simulink subsystem "MFTrailerTiresLongitudinal"  (R2023a)
settings: Solver=VariableStepAuto  StartTime=0.0  StopTime=10.0  RelTol=1e-3
libraries: autolibutils x1, autolibshared x1, autolibpowerinfoutils x1
(part 2 of 2)

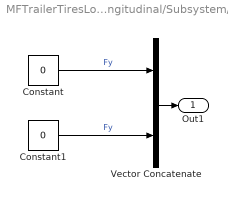
== system MFTrailerTiresLongitudinal/Subsystem/Fy ==
  Constant : Constant  Value=0  SampleTime=-1
  Constant1 : Constant  Value=0  SampleTime=-1
  Vector Concatenate : Concatenate
  Out1 : Outport  PortDimensions=2  VectorParamsAs1DForOutWhenUnconnected=off
  wires:
  Constant1/1 -> Vector Concatenate/2  "Fy"
  Vector Concatenate/1 -> Out1/1
  Constant/1 -> Vector Concatenate/1  "Fy"

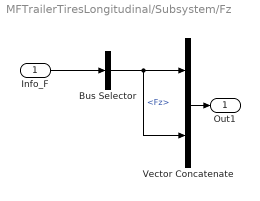
== system MFTrailerTiresLongitudinal/Subsystem/Fz ==
  Info_F : Inport
  Bus Selector : BusSelector  OutputSignals=Fz
  Vector Concatenate : Concatenate
  Out1 : Outport  PortDimensions=2  VectorParamsAs1DForOutWhenUnconnected=off
  wires:
  Vector Concatenate/1 -> Out1/1
  Info_F/1 -> Bus Selector/1
  Bus Selector/1 -> Vector Concatenate/1, Vector Concatenate/2  "<Fz>"

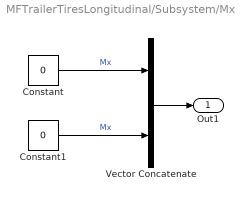
== system MFTrailerTiresLongitudinal/Subsystem/Mx ==
  Constant : Constant  Value=0  SampleTime=-1
  Constant1 : Constant  Value=0  SampleTime=-1
  Vector Concatenate : Concatenate
  Out1 : Outport  PortDimensions=2  VectorParamsAs1DForOutWhenUnconnected=off
  wires:
  Constant/1 -> Vector Concatenate/1  "Mx"
  Constant1/1 -> Vector Concatenate/2  "Mx"
  Vector Concatenate/1 -> Out1/1

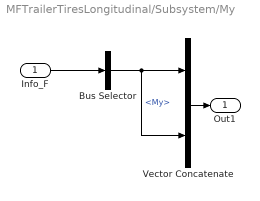
== system MFTrailerTiresLongitudinal/Subsystem/My ==
  Info_F : Inport
  Bus Selector : BusSelector  OutputSignals=My
  Vector Concatenate : Concatenate
  Out1 : Outport  PortDimensions=2  VectorParamsAs1DForOutWhenUnconnected=off
  wires:
  Bus Selector/1 -> Vector Concatenate/1, Vector Concatenate/2  "<My>"
  Info_F/1 -> Bus Selector/1
  Vector Concatenate/1 -> Out1/1

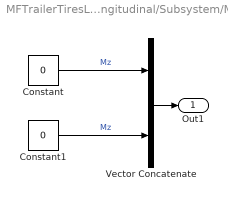
== system MFTrailerTiresLongitudinal/Subsystem/Mz ==
  Constant : Constant  Value=0  SampleTime=-1
  Constant1 : Constant  Value=0  SampleTime=-1
  Vector Concatenate : Concatenate
  Out1 : Outport  PortDimensions=2  VectorParamsAs1DForOutWhenUnconnected=off
  wires:
  Constant/1 -> Vector Concatenate/1  "Mz"
  Constant1/1 -> Vector Concatenate/2  "Mz"
  Vector Concatenate/1 -> Out1/1

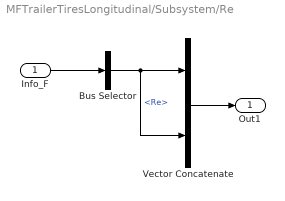
== system MFTrailerTiresLongitudinal/Subsystem/Re ==
  Info_F : Inport
  Bus Selector : BusSelector  OutputSignals=Re
  Vector Concatenate : Concatenate
  Out1 : Outport  PortDimensions=2  VectorParamsAs1DForOutWhenUnconnected=off
  wires:
  Vector Concatenate/1 -> Out1/1
  Info_F/1 -> Bus Selector/1
  Bus Selector/1 -> Vector Concatenate/1, Vector Concatenate/2  "<Re>"

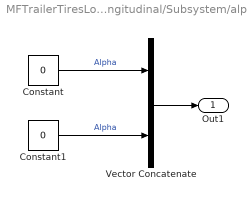
== system MFTrailerTiresLongitudinal/Subsystem/alpha ==
  Constant : Constant  Value=0  SampleTime=-1
  Constant1 : Constant  Value=0  SampleTime=-1
  Vector Concatenate : Concatenate
  Out1 : Outport  PortDimensions=2  VectorParamsAs1DForOutWhenUnconnected=off
  wires:
  Constant/1 -> Vector Concatenate/1  "Alpha"
  Constant1/1 -> Vector Concatenate/2  "Alpha"
  Vector Concatenate/1 -> Out1/1

== system MFTrailerTiresLongitudinal/Subsystem/kappa ==
  Info_F : Inport
  Bus Selector : BusSelector  OutputSignals=Kappa
  Vector Concatenate : Concatenate
  Out1 : Outport  PortDimensions=2  VectorParamsAs1DForOutWhenUnconnected=off
  wires:
  Bus Selector/1 -> Vector Concatenate/1, Vector Concatenate/2  "<Kappa>"
  Info_F/1 -> Bus Selector/1
  Vector Concatenate/1 -> Out1/1

== system MFTrailerTiresLongitudinal/Subsystem/omega ==
  Info_F : Inport
  Bus Selector : BusSelector  OutputSignals=Omega
  Vector Concatenate : Concatenate
  Out1 : Outport  PortDimensions=2  VectorParamsAs1DForOutWhenUnconnected=off
  wires:
  Info_F/1 -> Bus Selector/1
  Bus Selector/1 -> Vector Concatenate/1, Vector Concatenate/2  "<Omega>"
  Vector Concatenate/1 -> Out1/1

== system MFTrailerTiresLongitudinal/Subsystem/z ==
  Info_F : Inport
  Bus Selector : BusSelector  OutputSignals=z
  Vector Concatenate : Concatenate
  Out1 : Outport  PortDimensions=2  VectorParamsAs1DForOutWhenUnconnected=off
  wires:
  Bus Selector/1 -> Vector Concatenate/2, Vector Concatenate/1  "<z>"
  Info_F/1 -> Bus Selector/1
  Vector Concatenate/1 -> Out1/1

== system MFTrailerTiresLongitudinal/Subsystem/zdot ==
  Info_F : Inport
  Bus Selector : BusSelector  OutputSignals=zdot
  Vector Concatenate : Concatenate
  Out1 : Outport  PortDimensions=2  VectorParamsAs1DForOutWhenUnconnected=off
  wires:
  Vector Concatenate/1 -> Out1/1
  Info_F/1 -> Bus Selector/1
  Bus Selector/1 -> Vector Concatenate/1, Vector Concatenate/2  "<zdot>"
